simulink model "DCMachine"  (R2021b)
settings: Solver=VariableStepAuto  StartTime=0.0  StopTime=5  RelTol=1e-3
values from neighbouring files (symbols this model uses):
  B = 6.03e-6    (= 6.03e-06)    [DCMachine_cal.m]    (also in DC_Motor_speed_current_ctrl_cal.m = 0)
  J = 1.06e-6    (= 1.06e-06)    [DCMachine_cal.m]    (also in DC_Motor_speed_current_ctrl_cal.m = 0.156)
  Kphi = 1.41e-2    (= 0.0141)    [DCMachine_cal.m]    (also in DC_Motor_speed_current_ctrl_cal.m = 1.18236661951)
  La = 120e-3    (= 0.12)    [DCMachine_cal.m]    (also in DC_Motor_speed_current_ctrl_cal.m = 0.00293)
  Ra = 7    [DCMachine_cal.m]    (also in DC_Motor_speed_current_ctrl_cal.m = 0.18)
  Tl = 3.53e-3    (= 0.00353)    [DCMachine_cal.m]
  Vt = 6    [DCMachine_cal.m]    (also in DC_Motor_speed_current_ctrl_cal.m = 230)
Description:
  | The last lecture 11 exercise
settings Model: Creator=Dinh-Tuyen Le  LastModifiedBy=Dinh-Tuyen Le

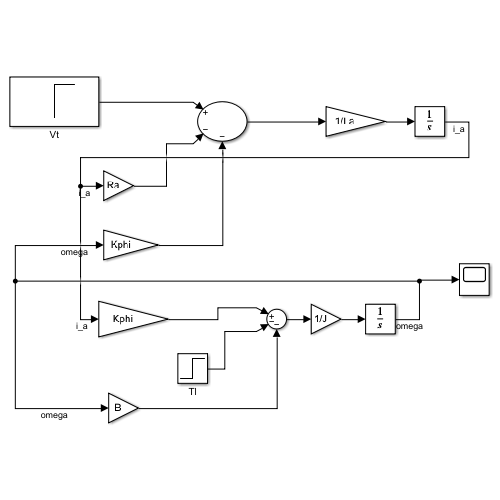
[thumbnail: Simulink's stored preview of the top-level diagram]
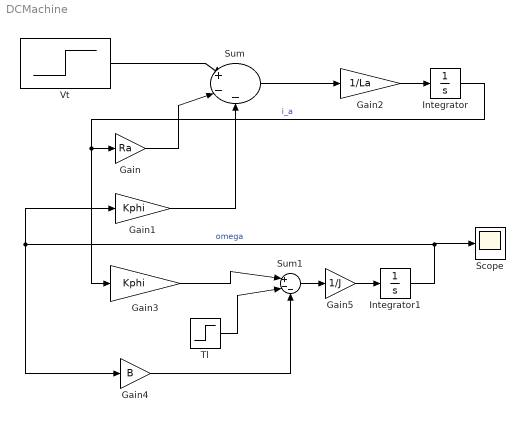
== system DCMachine ==
  Gain : Gain  Gain=Ra
  Gain1 : Gain  Gain=Kphi
  Gain2 : Gain  Gain=1/La
  Gain3 : Gain  Gain=Kphi
  Gain4 : Gain  Gain=B
  Gain5 : Gain  Gain=1/J
  Integrator : Integrator
  Integrator1 : Integrator
  Scope : Scope
  Sum : Sum  Inputs=|+--
  Sum1 : Sum  Inputs=|+--
  Tl : Step  Time=0  After=Tl  SampleTime=0
  Vt : Step  Time=0  After=Vt  SampleTime=0
  wires:
  Vt/1 -> Sum/1
  Gain/1 -> Sum/2
  Integrator1/1 -> Scope/1, Gain1/1, Gain4/1  "omega"
  Gain1/1 -> Sum/3
  Sum/1 -> Gain2/1
  Gain2/1 -> Integrator/1
  Integrator/1 -> Gain3/1, Gain/1  "i_a"
  Gain3/1 -> Sum1/1
  Tl/1 -> Sum1/2
  Gain4/1 -> Sum1/3
  Sum1/1 -> Gain5/1
  Gain5/1 -> Integrator1/1
